simulink model "PID_circuit_simulation"  (R2017b)
settings: Solver=VariableStepAuto  StartTime=0.0  StopTime=10.0  RelTol=1e-3
libraries: fl_lib x37, nesl_utility x2, elec_lib x2
settings Model: Creator=bhajd  LastModifiedBy=bhajd

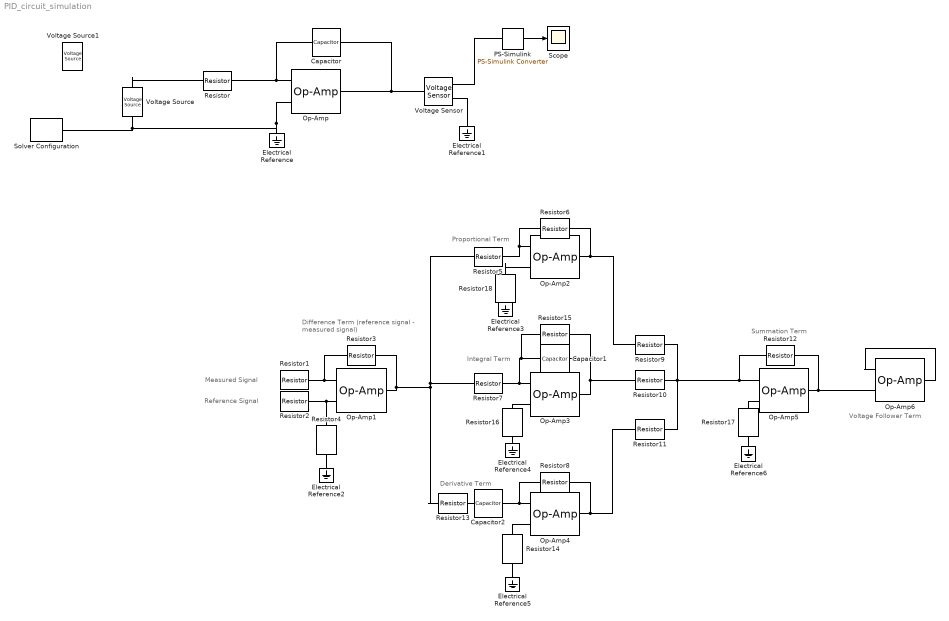
== system PID_circuit_simulation ==
  note: Reference Signal
  note: Proportional Term
  note: Integral Term
  note: Derivative Term
  note: Summation Term
  note: Voltage Follower Term
  note: Difference Term
      | (reference signal - measured signal)
  note: Measured Signal
  Capacitor : fl_lib/Electrical/Electrical Elements/Capacitor  c=1e-6 F  r=1e-6 Ohm  g=0 1/Ohm  i_specify=off  i_priority=None  i=0 A  i_nominal_specify=off  i_nominal_unit=A  i_nominal_value=1  v_specify=off  v_priority=None  v=0 V  v_nominal_specify=off  v_nominal_unit=V  v_nominal_value=1  vc_specify=off  vc_priority=High  vc=0 V  vc_nominal_specify=off  vc_nominal_unit=V  vc_nominal_value=1
  Capacitor1 : fl_lib/Electrical/Electrical Elements/Capacitor  c=1e-6 F  r=1e-6 Ohm  g=0 1/Ohm  i_specify=off  i_priority=None  i=0 A  i_nominal_specify=off  i_nominal_unit=A  i_nominal_value=1  v_specify=off  v_priority=None  v=0 V  v_nominal_specify=off  v_nominal_unit=V  v_nominal_value=1  vc_specify=off  vc_priority=High  vc=0 V  vc_nominal_specify=off  vc_nominal_unit=V  vc_nominal_value=1
  Capacitor2 : fl_lib/Electrical/Electrical Elements/Capacitor  c=1e-6 F  r=1e-6 Ohm  g=0 1/Ohm  i_specify=off  i_priority=None  i=0 A  i_nominal_specify=off  i_nominal_unit=A  i_nominal_value=1  v_specify=off  v_priority=None  v=0 V  v_nominal_specify=off  v_nominal_unit=V  v_nominal_value=1  vc_specify=off  vc_priority=High  vc=0 V  vc_nominal_specify=off  vc_nominal_unit=V  vc_nominal_value=1
  Electrical Reference{,1..6} (7 alike) : fl_lib/Electrical/Electrical Elements/Electrical Reference
  Op-Amp{,1..6} (7 alike) : fl_lib/Electrical/Electrical Elements/Op-Amp  outI_specify=off  outI_priority=None  outI=0 A  outI_nominal_specify=off  outI_nominal_unit=A  outI_nominal_value=1
  PS-Simulink : nesl_utility/PS-Simulink Converter  PhysicalDomain=network_engine_domain  SubClassName=ps_output  LeftPortType=input  RightPortType=output  PseudoPeriodic=off  Frequencies=[]  Unit=V  AffineConversion=off
  Resistor{,1..18} (19 alike) : fl_lib/Electrical/Electrical Elements/Resistor  R=1 Ohm  i_specify=off  i_priority=None  i=0 A  i_nominal_specify=off  i_nominal_unit=A  i_nominal_value=1  v_specify=off  v_priority=None  v=0 V  v_nominal_specify=off  v_nominal_unit=V  v_nominal_value=1
  Scope : Scope
  Solver Configuration : nesl_utility/Solver Configuration  PhysicalDomain=network_engine_domain  SubClassName=solver  LeftPortType=input  RightPortType=generic  Accelerate=off  Tones=[]  Harmonics=[]  SimulateNoise=off  Profile=off  UseLocalSampling=off  EnableSwitchedLinearOptims=on  FrequencyDomain=off  UseCCode=off  RelTol=0.001  AbsTol=1e-06  MinStep=1e-09  ToWorkspace=off  RevertToSquareIcSolve=off  NumHomotopyIterations=100  PhasorMode=off  PhasorModeNumHarmonics=1  DoDC=off  ResidualTolerance=1e-11  UseLocalSolver=off  LocalSolverChoice=NE_BACKWARD_EULER_ADVANCER  LocalSolverSampleTime=0.001  DoFixedCost=off  MaxNonlinIter=3  MaxModeIter=2  LinearAlgebra=Sparse  DelaysMemoryBudget=1024  AutomaticFiltering=on  FilteringTimeConstant=0.001
  Voltage Sensor : fl_lib/Electrical/Electrical Sensors/Voltage Sensor
  Voltage Source : elec_lib/Sources/Voltage Source  dc_voltage=0 V  ac_voltage=0 V  ac_shift=0 rad  ac_frequency=60 Hz  noise_mode=0  PSD=0 V^2/Hz  repeatability=1  auto_seed=2140457305  user_seed=0  sample_time=1e-3 s  i_specify=off  i_priority=None  i=0 A  i_nominal_specify=off  i_nominal_unit=A  i_nominal_value=1  v_specify=off  v_priority=None  v=0 V  v_nominal_specify=off  v_nominal_unit=V  v_nominal_value=1
      settings: SourceProductName=Simscape Electronics  SourceProductBaseCode=SN
  Voltage Source1 : elec_lib/Sources/Voltage Source  dc_voltage=0 V  ac_voltage=0 V  ac_shift=0 rad  ac_frequency=60 Hz  noise_mode=0  PSD=0 V^2/Hz  repeatability=1  auto_seed=3499211588  user_seed=0  sample_time=1e-3 s  i_specify=off  i_priority=None  i=0 A  i_nominal_specify=off  i_nominal_unit=A  i_nominal_value=1  v_specify=off  v_priority=None  v=0 V  v_nominal_specify=off  v_nominal_unit=V  v_nominal_value=1
      settings: SourceProductName=Simscape Electronics  SourceProductBaseCode=SN
  wires:
  PS-Simulink/1 -> Scope/1
  connections:
  Op-Amp/LConn1 -- Solver Configuration/RConn1 -- Voltage Source/RConn1 -- Electrical Reference/LConn1
  Resistor/RConn1 -- Capacitor/LConn1 -- Op-Amp/LConn2
  Capacitor/RConn1 -- Voltage Sensor/LConn1 -- Op-Amp/RConn1
  Voltage Source/LConn1 -- Resistor/LConn1
  Voltage Sensor/RConn1 -- PS-Simulink/LConn1
  Voltage Sensor/RConn2 -- Electrical Reference1/LConn1
  Electrical Reference2/LConn1 -- Resistor4/RConn1
  Resistor1/RConn1 -- Resistor3/LConn1 -- Op-Amp1/LConn2
  Resistor3/RConn1 -- Resistor13/LConn1 -- Resistor5/LConn1 -- Resistor7/LConn1 -- Op-Amp1/RConn1
  Resistor2/RConn1 -- Resistor4/LConn1 -- Op-Amp1/LConn1
  Capacitor1/LConn1 -- Resistor15/LConn1 -- Resistor7/RConn1 -- Op-Amp3/LConn2
  Resistor6/LConn1 -- Resistor5/RConn1 -- Op-Amp2/LConn2
  Capacitor2/RConn1 -- Resistor8/LConn1 -- Op-Amp4/LConn2
  Resistor8/RConn1 -- Resistor11/LConn1 -- Op-Amp4/RConn1
  Capacitor1/RConn1 -- Op-Amp3/RConn1 -- Resistor10/LConn1 -- Resistor15/RConn1
  Resistor6/RConn1 -- Resistor9/LConn1 -- Op-Amp2/RConn1
  Resistor9/RConn1 -- Resistor12/LConn1 -- Op-Amp5/LConn2 -- Resistor11/RConn1 -- Resistor10/RConn1
  Op-Amp6/LConn1 -- Resistor12/RConn1 -- Op-Amp5/RConn1
  Op-Amp6/LConn2 -- Op-Amp6/RConn1
  Resistor13/RConn1 -- Capacitor2/LConn1
  Resistor14/RConn1 -- Electrical Reference5/LConn1
  Resistor14/LConn1 -- Op-Amp4/LConn1
  Electrical Reference4/LConn1 -- Resistor16/RConn1
  Op-Amp3/LConn1 -- Resistor16/LConn1
  Resistor17/RConn1 -- Electrical Reference6/LConn1
  Op-Amp5/LConn1 -- Resistor17/LConn1
  Resistor18/LConn1 -- Op-Amp2/LConn1
